simulink model "Total_Pjt"  (R2025b)
settings: Solver=FixedStepDiscrete  StartTime=0.0  StopTime=inf  FixedStep=Ts  RelTol=1e-3
InitFcn:
  | para
values from neighbouring files (symbols this model uses):
  Ts = 0.01    [para.m]
settings Model: Creator=User  LastModifiedBy=User
settings OptimizationCC: DefaultParameterBehavior=Inlined  EnhancedBackFolding=on  PassReuseOutputArgsAs=Individual arguments  ZeroExternalMemoryAtStartup=off  ZeroInternalMemoryAtStartup=off  OptimizeBlockOrder=speed  DifferentSizesBufferReuse=on  OptimizationCustomize=off  EfficientTunableParamExpr=on
settings DebuggingCC: ParameterTunabilityLossMsg=error
settings HardwareCC: ProdBitPerPointer=32.0  ProdBitPerSizeT=32.0  ProdBitPerPtrDiffT=32.0  ProdLargestAtomicFloat=None  ProdWordSize=32.0  ProdHWDeviceType=Infineon->TriCore
settings SFSimCC: MATLABDynamicMemAlloc=off
settings RTWCC: SystemTargetFile=ert.tlc  GenCodeOnly=on  TemplateMakefile=ert_default_tmf  Description=Embedded Coder
settings CodeAppCC: ForceParamTrailComments=on  IgnoreCustomStorageClasses=off  OperatorAnnotations=on  SimulinkDataObjDesc=on  SFDataObjDesc=on  InsertBlockDesc=on
settings ERTTargetCC: ERTCustomFileTemplate=example_file_process.tlc  TargetLangStandard=C99 (ISO)  GenerateSampleERTMain=on

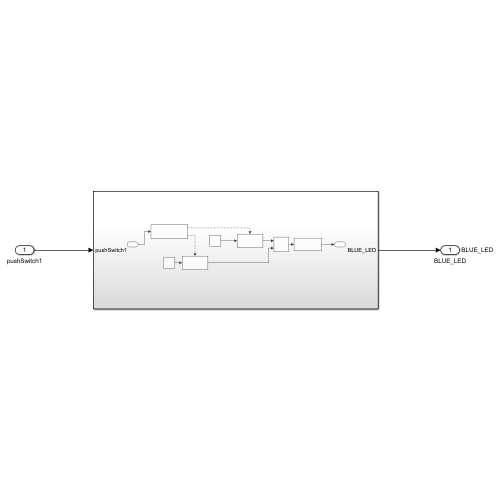
[thumbnail: Simulink's stored preview of the top-level diagram]
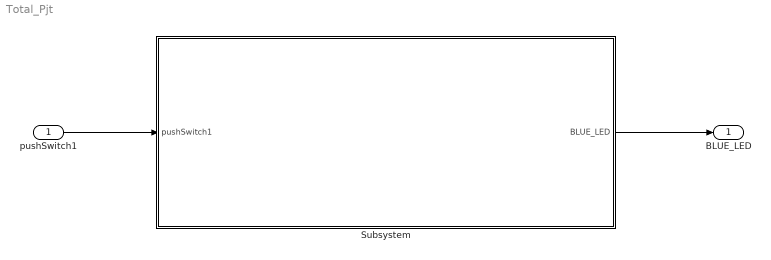
== system Total_Pjt ==
  pushSwitch1 : Inport  OutDataTypeStr=boolean
  Subsystem : Subsystem
  BLUE_LED : Outport  SignalName=BLUE_LED  OutMin=0  OutMax=50000  OutDataTypeStr=uint16
  wires:
  pushSwitch1/1 -> Subsystem/1(pushSwitch1)
  Subsystem/1(BLUE_LED) -> BLUE_LED/1

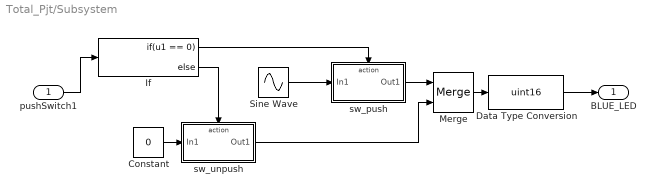
== system Total_Pjt/Subsystem ==
  pushSwitch1 : Inport
  Constant : Constant  Value=0
  Data Type Conversion : DataTypeConversion  OutDataTypeStr=uint16  SaturateOnIntegerOverflow=off  RndMeth=Floor
  If : If  IfExpression=u1 == 0
  Merge : Merge
  Sine Wave : Sin  SineType=Sample based  Amplitude=25000  Bias=25000  Samples=300  SampleTime=Ts
  "sw_push " : Subsystem  TreatAsAtomicUnit=on
  sw_unpush : Subsystem  TreatAsAtomicUnit=on
  BLUE_LED : Outport
  wires:
  pushSwitch1/1 -> If/1
  If/1 -> "sw_push "/Action
  If/2 -> sw_unpush/Action
  Constant/1 -> sw_unpush/1(In1)
  Sine Wave/1 -> "sw_push "/1(In1)
  "sw_push "/1(Out1) -> Merge/1
  sw_unpush/1(Out1) -> Merge/2
  Merge/1 -> Data Type Conversion/1
  Data Type Conversion/1 -> BLUE_LED/1

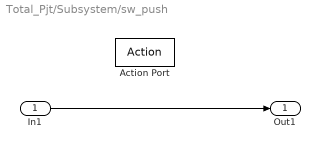
== system Total_Pjt/Subsystem/sw_push  ==
  In1 : Inport
  Action Port : ActionPort  ActionPortLabel=if(u1 == 0)
  Out1 : Outport
  wires:
  In1/1 -> Out1/1

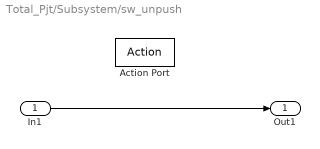
== system Total_Pjt/Subsystem/sw_unpush ==
  In1 : Inport
  Action Port : ActionPort  ActionPortLabel=else
  Out1 : Outport
  wires:
  In1/1 -> Out1/1
